simulink model "untitled"  (R2023b)
settings: Solver=VariableStepAuto  StartTime=0.0  StopTime=tsim  RelTol=1e-3
values from neighbouring files (symbols this model uses):
  Cz = (a1-zc)/b0    [artigoBismark.m]
  denFr = [1 -2*alpha alpha^2]    [artigoBismark.m]
  denGz = cell2mat(Gz.Denominator)    [artigoBismark.m]
  denSz = cell2mat(Sz.Denominator)    [artigoBismark.m]
  dn = 20    [artigoBismark.m]
  Fz = (1-zc)/(a1-zc)    [artigoBismark.m]
  numFr = [b1 b2 0]    [artigoBismark.m]
  numGz = cell2mat(Gz.Numerator)    [artigoBismark.m]
  numSz = cell2mat(Sz.Numerator)    [artigoBismark.m]
  Ts = 0.5    [artigoBismark.m]
settings Model: Creator=klysm  LastModifiedBy=klysm

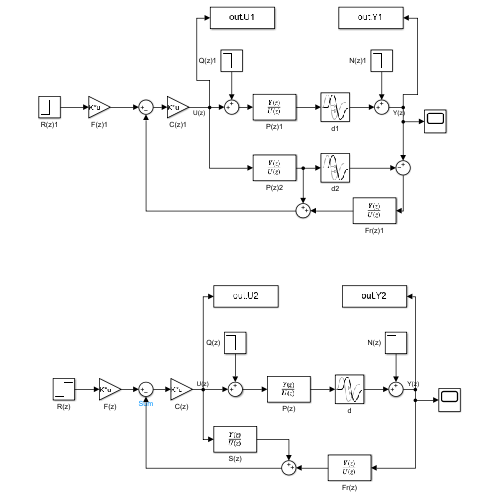
[thumbnail: Simulink's stored preview of the top-level diagram]
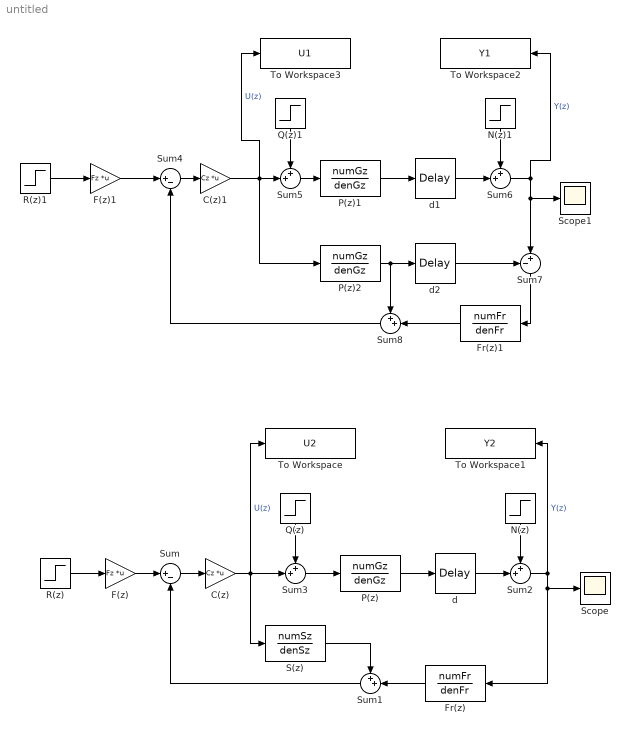
== system untitled ==
  C(z) : Gain  Gain=Cz  Multiplication=Matrix(K*u)
  C(z)1 : Gain  Gain=Cz  Multiplication=Matrix(K*u)
  F(z) : Gain  Gain=Fz  Multiplication=Matrix(K*u)
  F(z)1 : Gain  Gain=Fz  Multiplication=Matrix(K*u)
  Fr(z) : DiscreteTransferFcn  Numerator=numFr  Denominator=denFr
  Fr(z)1 : DiscreteTransferFcn  Numerator=numFr  Denominator=denFr
  N(z) : Step  Time=600  After=-1  SampleTime=Ts
  N(z)1 : Step  Time=600  After=-1  SampleTime=Ts
  P(z) : DiscreteTransferFcn  Numerator=numGz  Denominator=denGz
  P(z)1 : DiscreteTransferFcn  Numerator=numGz  Denominator=denGz
  P(z)2 : DiscreteTransferFcn  Numerator=numGz  Denominator=denGz
  Q(z) : Step  Time=200  After=-1  SampleTime=Ts
  Q(z)1 : Step  Time=200  After=-1  SampleTime=Ts
  R(z) : Step  Time=0  After=5  SampleTime=Ts
  R(z)1 : Step  Time=0  After=5  SampleTime=Ts
  S(z) : DiscreteTransferFcn  Numerator=numSz  Denominator=denSz
  Scope : Scope
  Scope1 : Scope
  Sum : Sum  Inputs=|+-
  Sum{1..3,5..6,8} (6 alike) : Sum  Inputs=++|
  Sum4 : Sum  Inputs=|+-
  Sum7 : Sum  Inputs=-+|
  To Workspace : ToWorkspace  VariableName=U2  SaveFormat=Timeseries  SampleTime=-1
  To Workspace1 : ToWorkspace  VariableName=Y2  SaveFormat=Timeseries  SampleTime=-1
  To Workspace2 : ToWorkspace  VariableName=Y1  SaveFormat=Timeseries  SampleTime=-1
  To Workspace3 : ToWorkspace  VariableName=U1  SaveFormat=Timeseries  SampleTime=-1
  d : TransportDelay  DelayTime=dn
  d1 : TransportDelay  DelayTime=dn
  d2 : TransportDelay  DelayTime=dn
  wires:
  F(z)/1 -> Sum/1
  R(z)/1 -> F(z)/1
  Q(z)/1 -> Sum3/1
  N(z)/1 -> Sum2/1
  Sum2/1 -> Scope/1, Fr(z)/1, To Workspace1/1  "Y(z)"
  Sum3/1 -> P(z)/1
  P(z)/1 -> d/1
  Sum/1 -> C(z)/1
  C(z)/1 -> To Workspace/1, S(z)/1, Sum3/2  "U(z)"
  S(z)/1 -> Sum1/1
  Fr(z)/1 -> Sum1/2
  Sum1/1 -> Sum/2
  d/1 -> Sum2/2
  R(z)1/1 -> F(z)1/1
  Sum4/1 -> C(z)1/1
  d1/1 -> Sum6/2
  P(z)1/1 -> d1/1
  Sum5/1 -> P(z)1/1
  N(z)1/1 -> Sum6/1
  C(z)1/1 -> To Workspace3/1, P(z)2/1, Sum5/2  "U(z)"
  Q(z)1/1 -> Sum5/1
  P(z)2/1 -> Sum8/1, d2/1
  d2/1 -> Sum7/1
  Sum6/1 -> Sum7/2, Scope1/1, To Workspace2/1  "Y(z)"
  Sum7/1 -> Fr(z)1/1
  Fr(z)1/1 -> Sum8/2
  Sum8/1 -> Sum4/2
  F(z)1/1 -> Sum4/1
